simulink model "ROS2_simulink_UE5_260106"  (R2024b)
settings: Solver=FixedStepAuto  StartTime=0.0  StopTime=1e6  FixedStep=0.1  RelTol=1e-3
model workspace (MAT data in the model file):
  SL_ROS_VariableLengthArrays_MaxSizes : object (value not decoded)
undefined symbols (not defined in the file): Aw_pont, B, B_pont, Cb_pont, coder, data, data_SL_Info, dt, Earth, encoding, height, I_L, I_T, IC, Ig_CG, k_neg, k_pos, L, l1, l2, LCF, m, rg, ros, Sim3dSensor, T_yaw, trim_setpoint, u_bp, Umax, WGS84, width, x, Xu_tab, y, z
libraries: ros2lib x13, sim3dlib x12, matrix_library x8, sharedutil x7, uavsimlib x6, simulink x4, simulink_extras x4, sharedtransform x3, visionsources x2, robotcorelib x1, aerolibtransform2 x1, sim3dcameralib x1
(part 3 of 3)

== matlab function ROS2_simulink_UE5_260106/Subsystem/Vessel Platform/Waves and Crossflow/Compute tau_crossflow ==
  data: L input; B input; T input; tau_crossflow output; nu_r input; rho input
function tau_crossflow = crossFlowDrag(L, B, T, nu_r, rho)

% tau_crossflow = crossFlowDrag(L,B,T,nu_r) computes the cross-flow drag 
% integrals for a marine craft using strip theory. Application:
%
%  M d/dt nu_r + C(nu_r)*nu_r + D*nu_r + g(eta) = tau + tau_crossflow
%
% Inputs: L:  length
%         B:  beam
%         T:  draft 
%         nu_r = [u-u_c, v-v_c, w-w_c, p, q, r]': relative velocity vector
%
% Output: tau_crossflow = [0 Yh 0 0 0 Nh]:  cross-flow drag in sway and yaw
%
% Author:     Thor I. Fossen 
% Date:       25 Apr 2021
% Revisions:  

% rho = 1026;             % density of water
n = 20;                 % number of strips

dx = L/20;             
Cd_2D = Hoerner(B,T);   % 2D drag coefficient based on Hoerner's curve

Yh = 0;
Nh = 0;
for xL = -L/2:dx:L/2
    v_r = nu_r(2);          % relative sway velocity
    r = nu_r(6);            % yaw rate
    Ucf = abs(v_r + xL * r) * (v_r + xL * r);
    Yh = Yh - 0.5 * rho * T * Cd_2D * Ucf * dx;         % sway force
    Nh = Nh - 0.5 * rho * T * Cd_2D * xL * Ucf * dx;    % yaw moment
end

tau_crossflow = [0 Yh 0 0 0 Nh]';

end

function CY_2D = Hoerner(B,T)
% Hoerner computes the 2D Hoerner cross-flow form coeff. as a function of B and T.
% he data is digizied and interpolation is used to compute other data points 
% than those in the table
%
%  CY_2D = Hoerner(B,T)
%
% Output: 
%    CY_2D:    2D Hoerner cross-flow form coefficient
%
% Inputs:
%    T:      draft (m)
%    B:      beam  (m)
%
% Author: Thor I. Fossen
% Date:   2007-12-01
%
% Reference:
% A. J. P. Leite, J. A. P. Aranha, C. Umeda and M. B. conti (1998). 
% Current force in tankers and bifurcation of equilibrium of turret
% systems: hydrodynamic model and experiments. 
% Applied Ocean Research 20, pp. 145-256.

% CD_DATA = [B/2T  C_D]
CD_DATA = [...    
0.0108623 1.96608
0.176606 1.96573
0.353025 1.89756
0.451863 1.78718
0.472838 1.58374
0.492877 1.27862
0.493252 1.21082
0.558473 1.08356
0.646401 0.998631
0.833589 0.87959
0.988002 0.828415
1.30807 0.759941
1.63918 0.691442
1.85998 0.657076
2.31288 0.630693
2.59998 0.596186
3.00877 0.586846
3.45075 0.585909
3.7379 0.559877
4.00309 0.559315];

CY_2D = interp1(CD_DATA(:,1),CD_DATA(:,2),B/(2*T),'linear','extrap');
ratio = B/(2*T);
if ratio < min(CD_DATA(:,1)) || ratio > max(CD_DATA(:,1))
    warning('B/(2T) = %.4f is outside data range. Using extrapolation.', ratio);
end
end

== matlab function ROS2_simulink_UE5_260106/simulink2UE1/MATLAB Function ==
  data: u1 input; y output; u2 input; u3 input
function y = fcn(u1, u2, u3)
u1 = u1*100 -2530.0; % unit in UE5: cm
u2 = u2*100 + 16720.0;
%#codegen
% 将三个标量信号拼成一个 [1x3] 行向量
y = [u1, u2, u3];

== matlab function ROS2_simulink_UE5_260106/simulink2UE1/MATLAB Function1 ==
  data: u1 input; y output; u2 input; u3 input
function y = fcn(u1, u2, u3)
%#codegen
% 将三个标量信号拼成一个 [1x3] 行向量
y = [u1, u2, u3];

== matlab function ROS2_simulink_UE5_260106/Subsystem/Vessel Platform/Thrust/MATLAB Function ==
  data: n_sig input; T_N output
function T_N = rpm2thrust(n_sig)
% n_sig: 转速信号 (rpm 向量或标量都可以)
% 输出: 推力 (N)，与输入维度一致

A = 8.18448e-05;   % kN / rpm^q
q = 2.17020;

% 如输入是 rad/s，请把下一行打开；如本来就是 rpm，则保持注释
% n_sig = n_sig * 60/(2*pi);  % rad/s -> rpm

% 幂律关系
TkN = sign(n_sig) .* (abs(n_sig).^q) * A;   % 单位: kN
T_N = 1000 * TkN;                           % 转换为 N

% -------- 低速死区处理 (逐元素) --------
% 建立逻辑索引，找到绝对值小于阈值的元素
idx = abs(n_sig) < 1e-3;
T_N(idx) = 0;

== matlab function ROS2_simulink_UE5_260106/MATLAB Function ==
  data: img_matrix input; height output; width output; encoding output; step output; data output; currentLength output
% function [height, width, encoding, step, data,currentLength] = createROS2ImageMsg(img_matrix)
%     [h, w, channels] = size(img_matrix);
% 
%     height = uint32(h);
%     width = uint32(w);
%     step = uint32(w * channels);
% 
%     % encoding 字符串 (128字节)
%     encoding = uint8(zeros(128, 1));
%     enc_str = 'rgb8';
%     encoding(1:length(enc_str)) = uint8(enc_str);
% 
%     % data (30000字节，注意是列向量)
%     data = uint8(reshape(img_matrix, [], 1));  % 列向量！
%     currentLength = numel(data);
% end


function [height, width, encoding, step, data, currentLength] = createROS2ImageMsg(img_matrix)
%#codegen

[h, w, channels] = size(img_matrix);

% 基本字段
height = uint32(h);
width = uint32(w);
step = uint32(w * channels);

% encoding 字符串
% % 创建足够大的 uint8 数组（例如 128）
% encoding = uint8(zeros(128, 1));
% 
% % 赋值并在尾部放一个字符终止符
% enc_str = 'rgb8';
% bytes = uint8([enc_str 0]); % 在末尾加 '\0'
% encoding(1:length(bytes)) = bytes;
encoding = 'rgb8';


% data 列向量
dataArray = uint8(reshape(img_matrix, [], 1)); 

% 把 data 和它的 CurrentLength 信息返回
data = dataArray;
currentLength = uint32(numel(dataArray));  

end
